simulink model "COMP_SYS_earth_checkered"  (R2026b)
settings: Solver=VariableStepAuto
undefined symbols (not defined in the file or in its folder): X, Y, Z
libraries: sm_lib x145
(part 1 of 19)
settings Model: Creator=bhorton  LastModifiedBy=bhorton
settings RTWCC: GPUComputeCapability=5.0

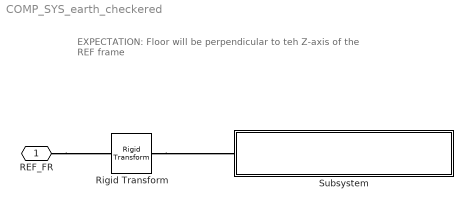
== system COMP_SYS_earth_checkered ==
  note: EXPECTATION:
      | Floor will be perpendicular to teh Z-axis of the REF frame
  Rigid Transform : sm_lib/Frames and Transforms/Rigid Transform  RotationMethod=None  FollAlignAxisA=+X  BaseAlignAxisA=+Y  FollAlignAxisB=+Y  BaseAlignAxisB=+Z  RotationStandardAxis=+Z  RotationAngle=0  RotationAngleUnits=deg  RotationArbitraryAxis=[0 0 1]  RotationSequenceAxes=FollowerAxes  RotationSequence=XYX  RotationSequenceAngles=[0 0 0]  RotationSequenceAnglesUnits=deg  RotationMatrix=[1 0 0;0 1 0;0 0 1]  Quaternion=[1 0 0 0]  TranslationMethod=Cartesian  TranslationCartesianOffset=earth_vis_OBJ.World_origin_of_SW_corner  TranslationCartesianOffsetUnits=m  TranslationStandardAxis=+Z  TranslationStandardOffset=0  TranslationStandardOffsetUnits=m  TranslationROffset=0  TranslationROffsetUnits=m  TranslationThetaOffset=0  TranslationThetaOffsetUnits=deg  TranslationZOffset=0  TranslationZOffsetUnits=m
  Subsystem : Subsystem
  REF_FR : PMIOPort  Side=Right
  connections:
  Rigid Transform/RConn1 -- Subsystem/LConn1
  REF_FR/RConn1 -- Rigid Transform/LConn1
